simulink model "spectrum_analyzer"  (R2023a)
settings: Solver=FixedStepDiscrete  StartTime=0.0  StopTime=inf  RelTol=1e-3  EnableMultiTasking=on
model workspace: external: MAT-File (data not in the file)
undefined symbols (not defined in the file or in its folder): daq
libraries: daqlib x1, dspspect3 x1
settings Model: Creator=The MathWorks, Inc.  LastModifiedBy=Administrator
settings SolverCC: AlgebraicLoopSolver=TrustRegion
settings DataIOCC: SaveFormat=Array  SaveOutput=off  SaveTime=off  ReturnWorkspaceOutputs=off  SignalLoggingName=logsOut
settings OptimizationCC: BlockReduction=off  BooleanDataType=off  InitFltsAndDblsToZero=on  LifeSpan=inf
settings DebuggingCC: SaveWithParameterizedLinksMsg=none  UnderspecifiedInitializationDetection=Classic  MergeDetectMultiDrivingBlocksExec=none  SignalResolutionControl=TryResolveAllWithWarning  MultiTaskDSMMsg=warning  MultiTaskCondExecSysMsg=none  FcnCallInpInsideContextMsg=warning  UnconnectedInputMsg=warning  UnconnectedOutputMsg=warning  UnconnectedLineMsg=warning  StateNameClashWarn=warning  SFUnexpectedBacktrackingDiag=warning  SFNoUnconditionalDefaultTransitionDiag=warning  SFExecutionAtInitializationDiag=none  ArithmeticOperatorsInVariantConditions=warning
settings HardwareCC: ProdBitPerPointer=32  ProdBitPerSizeT=32  ProdBitPerPtrDiffT=32  ProdLargestAtomicFloat=None  ProdIntDivRoundTo=Undefined  ProdEndianess=Unspecified  ProdWordSize=32  ProdHWDeviceType=Specified
settings ModelReferenceCC: EnableRefExpFcnMdlSchedulingChecks=on  PropagateSignalLabelsOutOfModel=off
settings SFSimCC: SimUseLocalCustomCode=off  CustomCodeUndefinedFunction=UseInterfaceOnly
settings RTWCC: RTWUseLocalCustomCode=off
settings CodeAppCC: StateflowObjectComments=on
settings GRTTargetCC: TargetFcnLib=ansi_tfl_tmw.mat  TargetLangStandard=C89/C90 (ANSI)  CombineOutputUpdateFcns=off  GRTInterface=on
settings ConfigComp: CovMetricSettings=d  CovSaveCumulativeToWorkspaceVar=on  CovSaveSingleToWorkspaceVar=on  CovExternalEMLEnable=off

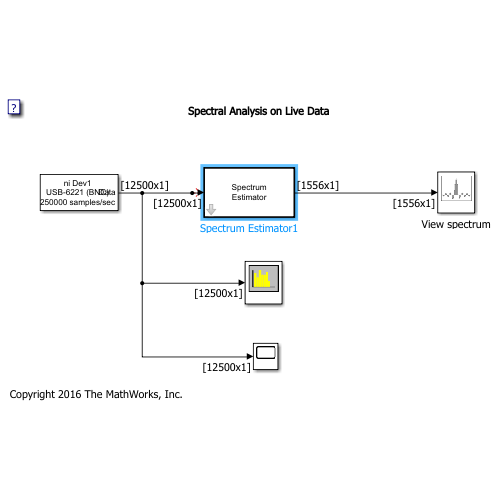
[thumbnail: Simulink's stored preview of the top-level diagram]
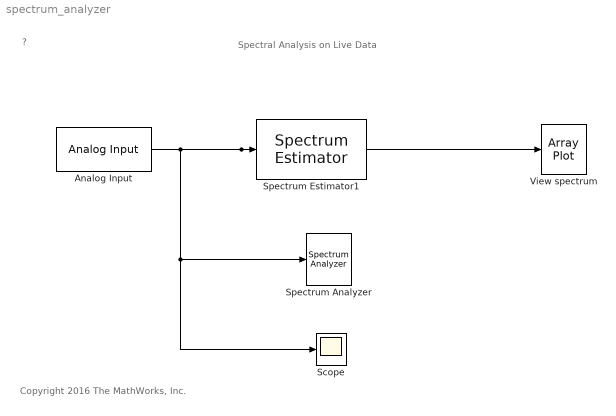
== system spectrum_analyzer ==
  note: Spectral Analysis on Live Data
  note: ?
  note: Copyright 2016 The MathWorks, Inc.
  Analog Input : daqlib/Analog Input  DeviceMenu=ni Dev1 (USB-6221 (BNC))  Device=ni Dev1 (USB-6221 (BNC))  ObjConstructor=daq.createSession('ni')  NChannelsSelected=1  Channels=1$ai0$$Dev1$1$4$3$1$#0$ai1$$Dev1$1$4$3$1$#0$ai2$$Dev1$1$4$3$1$#0$ai3$$Dev1$1$4$3$1$#0$ai4$$Dev1$1$4$3$1$#0$ai5$$Dev1$1$4$3$1$#0$ai6$$Dev1$1$4$3$1$#0$ai7$$Dev1$1$4$3$1$#0$ai8$$Dev1$1$4$1$1$#0$ai9$$Dev1$1$4$1$1$#0$ai10$$Dev1$1$4$1$1$#0$ai11$$Dev1$1$4$1$1$#0$ai12$$Dev1$1$4$1$1$#0$ai13$$Dev1$1$4$1$1$#0$ai14$$Dev1$1$4$1$1$#0$ai15$$Dev1$1$4$1$1$#  NPorts=1 for all channels  SampleRate=250000  ActualRate=250000  ScansPerTrigger=12500  OutputTimestamp=off  AcqMode=0  NumFrameBuffer=100  OutputTriggertime=off
  Scope : Scope
  Spectrum Analyzer : SpectrumAnalyzer  WindowPosition=[1.000000,41.000000,1536.000000,801.000000,]  ScopeFrameLocation=window  Method=Welch  Span=250000  StartFrequency=-125000  StopFrequency=125000  AveragingMethod=Running  YLimits=[-123.74351322,37.66547463]  ShowLegend=on
  Spectrum Estimator1 : dspspect3/Spectrum Estimator  Method=Welch  NumTapsPerBand=12  SpectrumType=Power  FrequencyResolutionMethod=Auto  FilterBankResolutionMethod=Auto  RBW=5  WindowLength=1024  FrequencyBandsSource=Same as input frame size  FrequencyBands=1024  FFTLengthSource=Auto  FFTLength=1024  InheritSampleRate=on  SampleRate=12500  Window=Chebyshev  SidelobeAttenuation=60  AveragingMethod=Running  SpectralAverages=1  ForgettingFactorPort=off  ForgettingFactor=0.9  Overlap=0  ReferenceLoad=50  FrequencyRange=One-sided  PowerUnits=dBm  SimulateUsing=Code generation  OutputMaxHoldSpectrum=off  OutputMinHoldSpectrum=off  OutputFrequencyVector=off  OutputRBW=off
  View spectrum : ArrayPlot  WindowPosition=[1.000000,41.000000,1536.000000,801.000000,]  ScopeFrameLocation=window  SampleIncrement=(10000)/(1024) / 1000  PlotType=Line  AxesScaling=Manual  XLabel=Frequency (KHz)  YLabel=dBm  YLimits=[-57.7228,17.1959]
  wires:
  Analog Input/1 -> Spectrum Estimator1/1, Scope/1, Spectrum Analyzer/1
  Spectrum Estimator1/1 -> View spectrum/1
